simulink model "VehiculoElectricoSimu"  (R2015a)
settings: Solver=ode45  StartTime=0.0  StopTime=10.0  RelTol=1e-3
values from neighbouring files (symbols this model uses):
  J = Jv+Jw+J1    (= 0.629243511638)    [VehiculoElectrico.m]
  Kbm = 1/((pi/30)*Kb)    (= 0.19098593171)    [VehiculoElectrico.m]
  Kpwm = 5    [VehiculoElectrico.m]
  Ktm = (0.1130)*Kt    (= 0.1808)    [VehiculoElectrico.m]
  La = 0.1e-3    (= 0.0001)    [VehiculoElectrico.m]
  n = 3    [VehiculoElectrico.m]
  Ra = 0.013    [VehiculoElectrico.m]
  Ts = 6.6666e-5    (= 6.6666e-05)    [VehiculoElectrico.m]
settings Model: Creator=luis_  LastModifiedBy=luis_

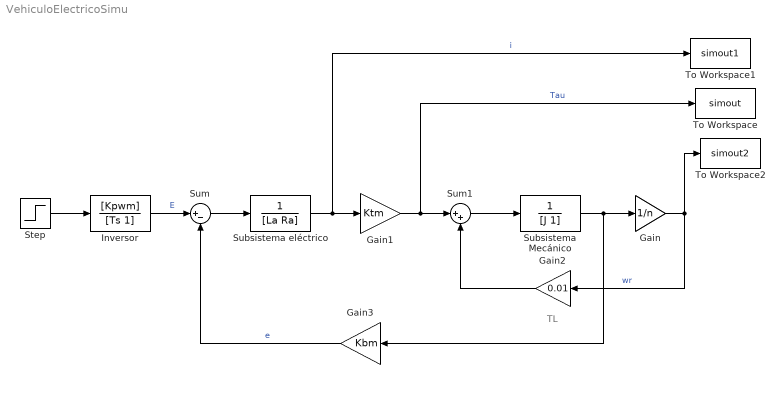
== system VehiculoElectricoSimu ==
  note: TL
  Gain : Gain  Gain=1/n
  Gain1 : Gain  Gain=Ktm
  Gain2 : Gain  Gain=0.01
  Gain3 : Gain  Gain=Kbm
  Inversor : TransferFcn  Numerator=[Kpwm]  Denominator=[Ts 1]
  Step : Step  After=70  SampleTime=0
  Subsistema Mecánico : TransferFcn  Denominator=[J 1]
  Subsistema eléctrico : TransferFcn  Denominator=[La Ra]
  Sum : Sum  Inputs=|+-
  Sum1 : Sum  Inputs=|++
  To Workspace : ToWorkspace  VariableName=simout  SaveFormat=Timeseries  SampleTime=-1
  To Workspace1 : ToWorkspace  VariableName=simout1  SaveFormat=Timeseries  SampleTime=-1
  To Workspace2 : ToWorkspace  VariableName=simout2  SaveFormat=Timeseries  SampleTime=-1
  wires:
  Sum1/1 -> Subsistema Mecánico/1
  Subsistema Mecánico/1 -> Gain3/1, Gain/1
  Gain/1 -> Gain2/1, To Workspace2/1  "wr"
  Step/1 -> Inversor/1
  Inversor/1 -> Sum/1  "E"
  Sum/1 -> Subsistema eléctrico/1
  Subsistema eléctrico/1 -> To Workspace1/1, Gain1/1  "i"
  Gain1/1 -> To Workspace/1, Sum1/1  "Tau"
  Gain3/1 -> Sum/2  "e"
  Gain2/1 -> Sum1/2
